simulink model "HarmonicDriveUr5_simulation"  (R2021a)
settings: Solver=ode15s  StartTime=0.0  StopTime=5  RelTol=1e-3
values from neighbouring files (symbols this model uses):
  K_lqr = lqr(A_c, B_c, Q, R)    [starterScript.m]
  Kd = 10    [starterScript.m]
  Ki = 2000    [starterScript.m]
  Kp = 40000    [starterScript.m]
  N = 100    [starterScript.m]
undefined symbols (not defined in the file or in its folder): X, Y, Z
libraries: fl_lib x60, sm_lib x57, nesl_utility x49, CustomComponents_lib x24, sdl_lib x6, roblocks x5
(part 1 of 3)
settings Model: Creator=agustin curri  LastModifiedBy=root
settings SolverCC: ZeroCrossAlgorithm=Adaptive  AlgebraicLoopSolver=TrustRegion
settings DebuggingCC: IgnoredZcDiagnostic=none  SFMachineParentedDataDiag=warning
settings ExplorerConfigSet: InternalSimMechanicsExplorerSettings="<ExplorerConfiguration><canonicalview>default</canonicalview><AnimationSetting><BasePlaybackSpeed>1.0</BasePlaybackSpeed><PlaybackSpeedFactor>1.0</PlaybackSpeedFactor></AnimationSetting><TilePanel><TileInfo><Tiles Columns=\"1\" Count=\"1\" Rows=\"1\"><Column Weight=\"1\"/><Row Weight=\"1\"/><Tile Height=\"1\" Width=\"1\" X=\"0\" Y=\"0\"/></Tiles></TileInfo><SceneInfo><SceneViewer><BGColor><R>1</R><G>1</G><B>1</B></BGColor><Camera><DoPerspective>off</DoPerspective><Position><X>0.024936801732020588</X><Y>-1.14355282845707174</Y><Z>0.464249949421630614</Z></Position><Center><X>0.024936801732020588</X><Y>-2.21862728744248727e-08</Y><Z>0.464249949421630614</Z></Center><Up><X>0</X><Y>-0</Y><Z>1</Z></Up><ViewLimDist>1</ViewLimDist><YLim>0.611217883330416378</YLim><XLim>1.22995074063620669</XLim></Camera></SceneViewer></SceneInfo></TilePanel><MechEditorPanel><Cameras/><GfxPanelCameraMap/><VideoCreator><PlaybackSpeedRatio>1.0</PlaybackSpeedRatio><FrameRate>30</FrameRate><VideoFormat>Motion JPEG AVI</VideoFormat><FrameSize>auto</FrameSize></VideoCreator></MechEditorPanel></ExplorerConfiguration>"

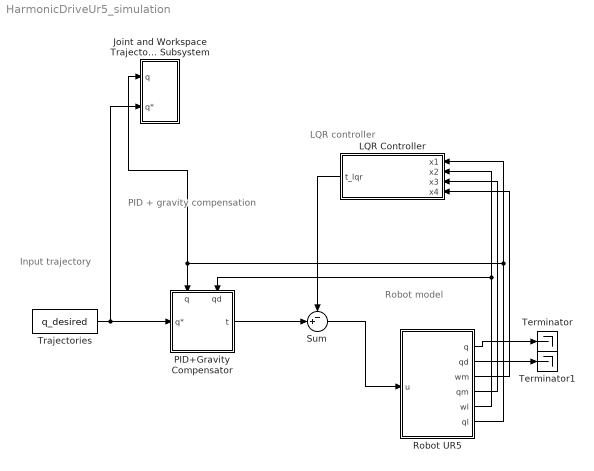
== system HarmonicDriveUr5_simulation ==
  note: Robot model
  note: LQR controller
  note: Input trajectory
  note: PID + gravity compensation
  Joint and Workspace Trajectory Subsystem : Subsystem
  LQR Controller : Subsystem
  PID+Gravity Compensator : Subsystem
      settings: PortSchema="{\"entries\":[{\"content\":{\"sides\":[{\"content\":{\"connectorIds\":[\"In1\"]},\"type\":\"ConnectorPlacement.EquallySpacedRectSide\",\"uuid\":\"10e36f8c-91af-4a0b-8edd-006e92f80377\"},{\"content\":{\"connectorIds\":[\"Out1\"],\"side\":\"RIGHT\"},\"type\":\"ConnectorPlacement.EquallySpacedRectSide\",\"uuid\":\"e975d4b2-2c07-4038-bb63-9e1fdc9bbfc2\"},{\"content\":{\"connectorIds\":[\"In2\",\"In3\"],\"side\":\"TOP\"},\"type\":\"ConnectorPlacement.EquallySpacedRectSide\",\"uuid\":\"401cadff-8190-4a51-9549-9161046c9efc\"}]},\"type\":\"ConnectorPlacement.EquallySpacedConnector\",\"uuid\":\"e3d6090e-dadc-41ed-ab00-96ae674af8f5\"}],\"packageUris\":[\"http://schema.mathworks.com/mf0/Connector/R2020b\"],\"version\":\"1.0\"}"
  Robot UR5 : Subsystem
  Sum : Sum  Inputs=-+|
  Terminator : Terminator
  Terminator1 : Terminator
  Trajectories : FromWorkspace  VariableName=q_desired
  wires:
  LQR Controller/1(t_lqr) -> Sum/1
  PID+Gravity Compensator/1(t) -> Sum/2
  Sum/1 -> Robot UR5/1(u)
  Trajectories/1 -> Joint and Workspace Trajectory Subsystem/2(q*), PID+Gravity Compensator/1(q*)
  Robot UR5/3(wm) -> LQR Controller/4(x4)
  Robot UR5/4(qm) -> LQR Controller/3(x3)
  Robot UR5/5(wl) -> PID+Gravity Compensator/3(qd), LQR Controller/2(x2)
  Robot UR5/6(ql) -> Joint and Workspace Trajectory Subsystem/1(q), PID+Gravity Compensator/2(q), LQR Controller/1(x1)
  Robot UR5/1(q) -> Terminator/1
  Robot UR5/2(qd) -> Terminator1/1

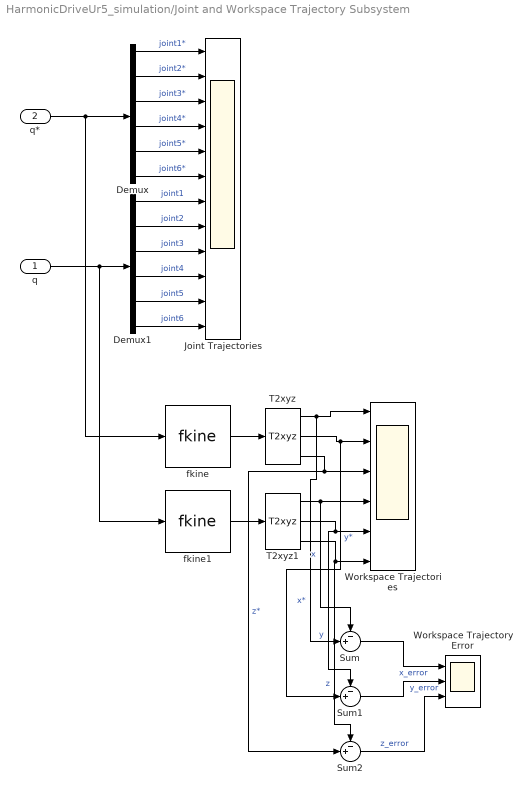
== system HarmonicDriveUr5_simulation/Joint and Workspace Trajectory Subsystem ==
  q : Inport
  q* : Inport  Port=2
  Demux : Demux  Outputs=6
  Demux1 : Demux  Outputs=6
  Joint Trajectories : Scope  NumInputPorts=12
  Sum : Sum  Inputs=-+|
  Sum1 : Sum  Inputs=-+|
  Sum2 : Sum  Inputs=-+|
  T2xyz : roblocks/Toolbox/T2xyz
  T2xyz1 : roblocks/Toolbox/T2xyz
  Workspace Trajectories : Scope  NumInputPorts=6
  Workspace Trajectory Error : Scope  NumInputPorts=3
  fkine : roblocks/Arm/fkine  robot=ur5
  fkine1 : roblocks/Arm/fkine  robot=ur5
  wires:
  Demux/4 -> Joint Trajectories/4  "joint4*"
  Demux1/2 -> Joint Trajectories/8  "joint2"
  Demux1/4 -> Joint Trajectories/10  "joint4"
  Demux1/6 -> Joint Trajectories/12  "joint6"
  Demux1/3 -> Joint Trajectories/9  "joint3"
  Demux/5 -> Joint Trajectories/5  "joint5*"
  Demux1/5 -> Joint Trajectories/11  "joint5"
  q*/1 -> fkine/1, Demux/1
  Demux/1 -> Joint Trajectories/1  "joint1*"
  q/1 -> fkine1/1, Demux1/1
  Demux1/1 -> Joint Trajectories/7  "joint1"
  Demux/6 -> Joint Trajectories/6  "joint6*"
  Demux/3 -> Joint Trajectories/3  "joint3*"
  Demux/2 -> Joint Trajectories/2  "joint2*"
  fkine/1 -> T2xyz/1
  T2xyz/1 -> Sum/2, Workspace Trajectories/1  "x*"
  T2xyz/2 -> Sum1/2, Workspace Trajectories/2  "y*"
  T2xyz/3 -> Workspace Trajectories/3, Sum2/2  "z*"
  fkine1/1 -> T2xyz1/1
  T2xyz1/1 -> Workspace Trajectories/4, Sum/1  "x"
  T2xyz1/2 -> Workspace Trajectories/5, Sum1/1  "y"
  T2xyz1/3 -> Workspace Trajectories/6, Sum2/1  "z"
  Sum/1 -> Workspace Trajectory Error/1  "x_error"
  Sum1/1 -> Workspace Trajectory Error/2  "y_error"
  Sum2/1 -> Workspace Trajectory Error/3  "z_error"

== system HarmonicDriveUr5_simulation/LQR Controller ==
  x1 : Inport
  x2 : Inport  Port=2
  x3 : Inport  Port=3
  x4 : Inport  Port=4
  MATLAB Function : MATLAB Function  TreatAsAtomicUnit=on  mask{K_lqr=K_lqr}
  Vector Concatenate : Concatenate  NumInputs=4
  t_lqr : Outport
  wires:
  x3/1 -> Vector Concatenate/3
  MATLAB Function/1(t) -> t_lqr/1
  Vector Concatenate/1 -> MATLAB Function/1(x)
  x1/1 -> Vector Concatenate/1
  x2/1 -> Vector Concatenate/2
  x4/1 -> Vector Concatenate/4

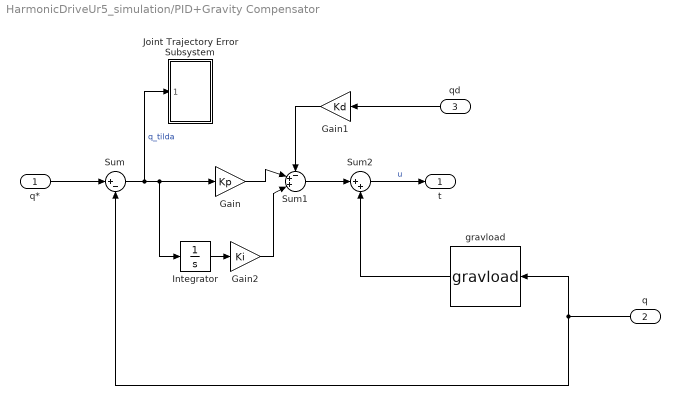
== system HarmonicDriveUr5_simulation/PID+Gravity Compensator ==
  q* : Inport
  q : Inport  Port=2
  qd : Inport  Port=3
  Gain : Gain  Gain=Kp
  Gain1 : Gain  Gain=Kd
  Gain2 : Gain  Gain=Ki
  Integrator : Integrator
  Joint Trajectory Error Subsystem : Subsystem
  Sum : Sum  Inputs=|+-
  Sum1 : Sum  Inputs=-++|
  Sum2 : Sum  Inputs=|++
  gravload : roblocks/Arm/gravload  robot=ur5
  t : Outport
  wires:
  Sum1/1 -> Sum2/1
  Sum/1 -> Joint Trajectory Error Subsystem/1(q_tilda), Gain/1, Integrator/1  "q_tilda"
  Gain2/1 -> Sum1/3
  qd/1 -> Gain1/1
  Integrator/1 -> Gain2/1
  q*/1 -> Sum/1
  q/1 -> gravload/1, Sum/2
  Gain1/1 -> Sum1/1
  Sum2/1 -> t/1  "u"
  Gain/1 -> Sum1/2
  gravload/1 -> Sum2/2

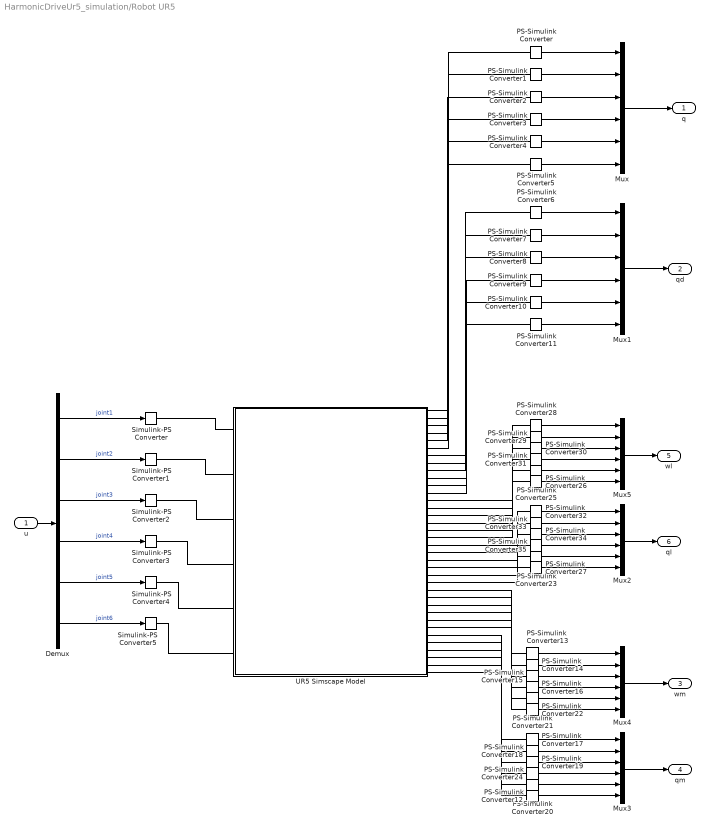
== system HarmonicDriveUr5_simulation/Robot UR5 ==
  u : Inport
  Demux : Demux  Outputs=6
  Mux{,1..5} (6 alike) : Mux  Inputs=6
  PS-Simulink Converter{,1..11} (12 alike) : nesl_utility/PS-Simulink Converter  PhysicalDomain=network_engine_domain  SubClassName=ps_output  LeftPortType=input  RightPortType=output  PseudoPeriodic=off  Frequencies=[]  Unit=inherit  AffineConversion=off
      settings: SourceProductBaseCode=PW,SS
  PS-Simulink Converter{12,17..20,23..24,27,32..35} (12 alike) : nesl_utility/PS-Simulink Converter  PhysicalDomain=network_engine_domain  SubClassName=ps_output  LeftPortType=input  RightPortType=output  PseudoPeriodic=off  Frequencies=[]  Unit=rad  AffineConversion=off
      settings: SourceProductBaseCode=PW,SS
  PS-Simulink Converter{13..16,21..22,25..26,28..31} (12 alike) : nesl_utility/PS-Simulink Converter  PhysicalDomain=network_engine_domain  SubClassName=ps_output  LeftPortType=input  RightPortType=output  PseudoPeriodic=off  Frequencies=[]  Unit=rad/s  AffineConversion=off
      settings: SourceProductBaseCode=PW,SS
  Simulink-PS Converter{,1..5} (6 alike) : nesl_utility/Simulink-PS Converter  PhysicalDomain=network_engine_domain  SubClassName=ps_input  LeftPortType=input  RightPortType=output  PseudoPeriodic=off  Frequencies=[]  NoiseDistribution=none  NoiseParameters=[]  Unit=1  AffineConversion=off  FilteringAndDerivatives=provide  SimscapeFilterOrder=2  InputFilterTimeConstant=0.001  UdotUserProvided=0
      settings: SourceProductBaseCode=PW,SS
  UR5 Simscape Model : Subsystem
  q : Outport
  qd : Outport  Port=2
  wm : Outport  Port=3
  qm : Outport  Port=4
  wl : Outport  Port=5
  ql : Outport  Port=6
  wires:
  Demux/6 -> Simulink-PS Converter5/1  "joint6"
  PS-Simulink Converter6/1 -> Mux1/1
  PS-Simulink Converter5/1 -> Mux/6
  PS-Simulink Converter7/1 -> Mux1/2
  PS-Simulink Converter8/1 -> Mux1/3
  u/1 -> Demux/1
  PS-Simulink Converter10/1 -> Mux1/5
  Demux/2 -> Simulink-PS Converter1/1  "joint2"
  PS-Simulink Converter4/1 -> Mux/5
  PS-Simulink Converter1/1 -> Mux/2
  PS-Simulink Converter/1 -> Mux/1
  Demux/1 -> Simulink-PS Converter/1  "joint1"
  Mux/1 -> q/1
  PS-Simulink Converter9/1 -> Mux1/4
  Mux1/1 -> qd/1
  Demux/5 -> Simulink-PS Converter4/1  "joint5"
  PS-Simulink Converter11/1 -> Mux1/6
  PS-Simulink Converter3/1 -> Mux/4
  Demux/4 -> Simulink-PS Converter3/1  "joint4"
  Demux/3 -> Simulink-PS Converter2/1  "joint3"
  PS-Simulink Converter2/1 -> Mux/3
  PS-Simulink Converter17/1 -> Mux3/1
  Mux3/1 -> qm/1
  PS-Simulink Converter18/1 -> Mux3/2
  PS-Simulink Converter14/1 -> Mux4/2
  PS-Simulink Converter15/1 -> Mux4/3
  PS-Simulink Converter13/1 -> Mux4/1
  PS-Simulink Converter21/1 -> Mux4/5
  PS-Simulink Converter24/1 -> Mux3/4
  PS-Simulink Converter20/1 -> Mux3/5
  PS-Simulink Converter12/1 -> Mux3/6
  PS-Simulink Converter19/1 -> Mux3/3
  PS-Simulink Converter22/1 -> Mux4/6
  PS-Simulink Converter16/1 -> Mux4/4
  Mux4/1 -> wm/1
  Mux5/1 -> wl/1
  PS-Simulink Converter26/1 -> Mux5/6
  PS-Simulink Converter29/1 -> Mux5/2
  PS-Simulink Converter31/1 -> Mux5/4
  PS-Simulink Converter25/1 -> Mux5/5
  Mux2/1 -> ql/1
  PS-Simulink Converter23/1 -> Mux2/5
  PS-Simulink Converter28/1 -> Mux5/1
  PS-Simulink Converter33/1 -> Mux2/2
  PS-Simulink Converter35/1 -> Mux2/4
  PS-Simulink Converter27/1 -> Mux2/6
  PS-Simulink Converter34/1 -> Mux2/3
  PS-Simulink Converter30/1 -> Mux5/3
  PS-Simulink Converter32/1 -> Mux2/1
  connections:
  UR5 Simscape Model/RConn1 -- PS-Simulink Converter/LConn1
  UR5 Simscape Model/RConn2 -- PS-Simulink Converter1/LConn1
  UR5 Simscape Model/RConn3 -- PS-Simulink Converter2/LConn1
  UR5 Simscape Model/RConn4 -- PS-Simulink Converter3/LConn1
  UR5 Simscape Model/RConn5 -- PS-Simulink Converter4/LConn1
  UR5 Simscape Model/RConn6 -- PS-Simulink Converter5/LConn1
  Simulink-PS Converter/RConn1 -- UR5 Simscape Model/LConn1
  UR5 Simscape Model/RConn7 -- PS-Simulink Converter6/LConn1
  Simulink-PS Converter1/RConn1 -- UR5 Simscape Model/LConn2
  UR5 Simscape Model/RConn8 -- PS-Simulink Converter7/LConn1
  Simulink-PS Converter2/RConn1 -- UR5 Simscape Model/LConn3
  UR5 Simscape Model/RConn9 -- PS-Simulink Converter8/LConn1
  Simulink-PS Converter3/RConn1 -- UR5 Simscape Model/LConn4
  UR5 Simscape Model/RConn10 -- PS-Simulink Converter9/LConn1
  Simulink-PS Converter4/RConn1 -- UR5 Simscape Model/LConn5
  UR5 Simscape Model/RConn11 -- PS-Simulink Converter10/LConn1
  Simulink-PS Converter5/RConn1 -- UR5 Simscape Model/LConn6
  UR5 Simscape Model/RConn12 -- PS-Simulink Converter11/LConn1
  UR5 Simscape Model/RConn25 -- PS-Simulink Converter13/LConn1
  UR5 Simscape Model/RConn26 -- PS-Simulink Converter14/LConn1
  UR5 Simscape Model/RConn27 -- PS-Simulink Converter15/LConn1
  UR5 Simscape Model/RConn28 -- PS-Simulink Converter16/LConn1
  UR5 Simscape Model/RConn29 -- PS-Simulink Converter21/LConn1
  UR5 Simscape Model/RConn30 -- PS-Simulink Converter22/LConn1
  UR5 Simscape Model/RConn31 -- PS-Simulink Converter17/LConn1
  UR5 Simscape Model/RConn32 -- PS-Simulink Converter18/LConn1
  UR5 Simscape Model/RConn33 -- PS-Simulink Converter19/LConn1
  UR5 Simscape Model/RConn34 -- PS-Simulink Converter24/LConn1
  UR5 Simscape Model/RConn35 -- PS-Simulink Converter20/LConn1
  UR5 Simscape Model/RConn36 -- PS-Simulink Converter12/LConn1
  UR5 Simscape Model/RConn13 -- PS-Simulink Converter28/LConn1
  UR5 Simscape Model/RConn14 -- PS-Simulink Converter29/LConn1
  UR5 Simscape Model/RConn15 -- PS-Simulink Converter30/LConn1
  UR5 Simscape Model/RConn16 -- PS-Simulink Converter31/LConn1
  UR5 Simscape Model/RConn17 -- PS-Simulink Converter25/LConn1
  UR5 Simscape Model/RConn18 -- PS-Simulink Converter26/LConn1
  UR5 Simscape Model/RConn19 -- PS-Simulink Converter32/LConn1
  UR5 Simscape Model/RConn20 -- PS-Simulink Converter33/LConn1
  UR5 Simscape Model/RConn21 -- PS-Simulink Converter34/LConn1
  UR5 Simscape Model/RConn22 -- PS-Simulink Converter35/LConn1
  UR5 Simscape Model/RConn23 -- PS-Simulink Converter23/LConn1
  UR5 Simscape Model/RConn24 -- PS-Simulink Converter27/LConn1

== system HarmonicDriveUr5_simulation/PID+Gravity Compensator/Joint Trajectory Error Subsystem ==
  q_tilda : Inport
  Demux : Demux  Outputs=6
  Joint Trajectory Error : Scope  NumInputPorts=6
  wires:
  Demux/5 -> Joint Trajectory Error/5  "joint5"
  q_tilda/1 -> Demux/1
  Demux/2 -> Joint Trajectory Error/2  "joint2"
  Demux/3 -> Joint Trajectory Error/3  "joint3"
  Demux/4 -> Joint Trajectory Error/4  "joint4"
  Demux/6 -> Joint Trajectory Error/6  "joint6"
  Demux/1 -> Joint Trajectory Error/1  "joint1"

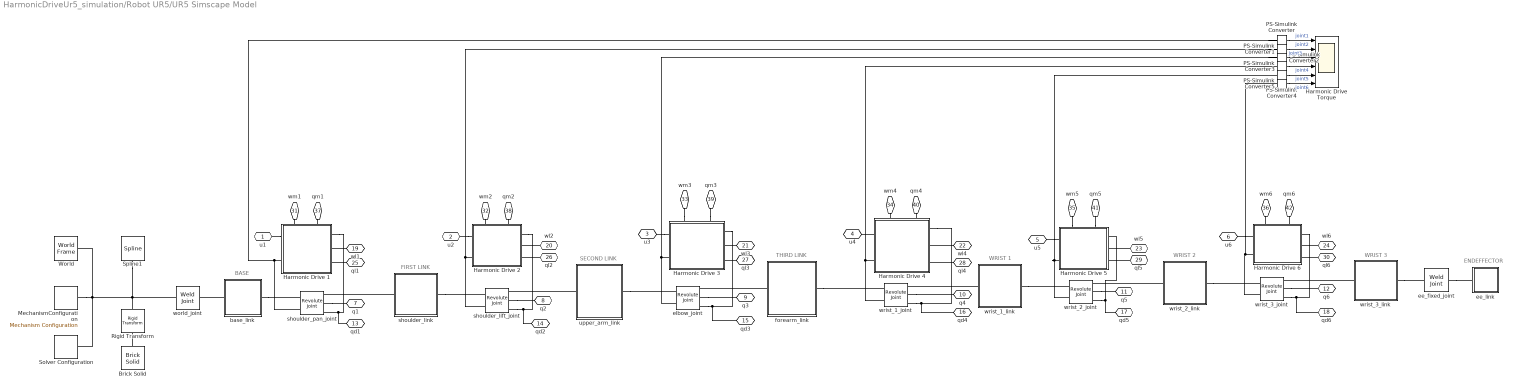
== system HarmonicDriveUr5_simulation/Robot UR5/UR5 Simscape Model ==
  note: BASE
  note: FIRST LINK
  note: SECOND LINK
  note: THIRD LINK
  note: WRIST 1
  note: WRIST 2
  note: WRIST 3
  note: ENDEFFECTOR
  Brick Solid : sm_lib/Body Elements/Brick Solid  GraphicAmbientColor=[0.15 0.15 0.15 1.0]  BasedOnType=Density  BrickDimensions=[.5 .5 0.2]  BrickDimensionUnits=m  CenterOfMass=[0 0 0]  CenterOfMassUnits=m  GraphicDiffuseColor=[0.8 1.0 0.6]  Density=1000  DensityUnits=kg/m^3  DoExposeReferenceFrame=on  GraphicEmissiveColor=[0.0 0.0 0.0 1.0]  ExportEntireGeometry=off  SerializedFrames=<Frames/>  MarkerShape=Sphere  MarkerSize=10  GraphicType=FromGeometry  InertiaType=CalculateFromGeometry  Mass=1  MassUnits=kg  MomentsOfInertia=[1 1 1]  MomentsOfInertiaUnits=kg*m^2  GraphicOpacity=1.0  ProductsOfInertia=[0 0 0]  ProductsOfInertiaUnits=kg*m^2  GraphicShininess=75  GraphicSpecularColor=[0.5 0.5 0.5 1.0]  GraphicVisPropType=SimpleVisualProperties
  Harmonic Drive 1 : Subsystem
      settings: PortSchema="{\"entries\":[{\"content\":{\"sides\":[{\"content\":{\"connectorIds\":[\"LConn1\",\"LConn2\"]},\"type\":\"ConnectorPlacement.EquallySpacedRectSide\",\"uuid\":\"507705ac-a0fa-4fe7-8f73-31050ecbd987\"},{\"content\":{\"connectorIds\":[\"RConn1\",\"RConn2\",\"RConn3\"],\"side\":\"RIGHT\"},\"type\":\"ConnectorPlacement.EquallySpacedRectSide\",\"uuid\":\"f13bfcdd-63e8-47b4-aefd-dba91edbc643\"},{\"content\":{\"connectorIds\":[\"LConn3\",\"LConn4\"],\"side\":\"TOP\"},\"type\":\"ConnectorPlacement.EquallySpacedRectSide\",\"uuid\":\"144ffa6a-f599-4bcb-ae05-6789f1cae58f\"}]},\"type\":\"ConnectorPlacement.EquallySpacedConnector\",\"uuid\":\"4d436d19-1cb5-4db6-9907-e987ea85be45\"}],\"packageUris\":[\"http://schema.mathworks.com/mf0/Connector/R2020b\"],\"version\":\"1.0\"}"
      mask Display: image('$imagefile'); % Use "Edit Image" on toolstrip to change.
  Harmonic Drive 2 : Subsystem
      settings: PortSchema="{\"entries\":[{\"content\":{\"sides\":[{\"content\":{\"connectorIds\":[\"LConn1\",\"LConn2\"]},\"type\":\"ConnectorPlacement.EquallySpacedRectSide\",\"uuid\":\"507705ac-a0fa-4fe7-8f73-31050ecbd987\"},{\"content\":{\"connectorIds\":[\"RConn1\",\"RConn2\",\"RConn3\"],\"side\":\"RIGHT\"},\"type\":\"ConnectorPlacement.EquallySpacedRectSide\",\"uuid\":\"f13bfcdd-63e8-47b4-aefd-dba91edbc643\"},{\"content\":{\"connectorIds\":[\"LConn3\",\"LConn4\"],\"side\":\"TOP\"},\"type\":\"ConnectorPlacement.EquallySpacedRectSide\",\"uuid\":\"144ffa6a-f599-4bcb-ae05-6789f1cae58f\"}]},\"type\":\"ConnectorPlacement.EquallySpacedConnector\",\"uuid\":\"4d436d19-1cb5-4db6-9907-e987ea85be45\"}],\"packageUris\":[\"http://schema.mathworks.com/mf0/Connector/R2020b\"],\"version\":\"1.0\"}"
      mask Display: image('$imagefile'); % Use "Edit Image" on toolstrip to change.
  Harmonic Drive 3 : Subsystem
      settings: PortSchema="{\"entries\":[{\"content\":{\"sides\":[{\"content\":{\"connectorIds\":[\"LConn1\",\"LConn2\"]},\"type\":\"ConnectorPlacement.EquallySpacedRectSide\",\"uuid\":\"507705ac-a0fa-4fe7-8f73-31050ecbd987\"},{\"content\":{\"connectorIds\":[\"RConn1\",\"RConn2\",\"RConn3\"],\"side\":\"RIGHT\"},\"type\":\"ConnectorPlacement.EquallySpacedRectSide\",\"uuid\":\"f13bfcdd-63e8-47b4-aefd-dba91edbc643\"},{\"content\":{\"connectorIds\":[\"LConn3\",\"LConn4\"],\"side\":\"TOP\"},\"type\":\"ConnectorPlacement.EquallySpacedRectSide\",\"uuid\":\"144ffa6a-f599-4bcb-ae05-6789f1cae58f\"}]},\"type\":\"ConnectorPlacement.EquallySpacedConnector\",\"uuid\":\"4d436d19-1cb5-4db6-9907-e987ea85be45\"}],\"packageUris\":[\"http://schema.mathworks.com/mf0/Connector/R2020b\"],\"version\":\"1.0\"}"
      mask Display: image('$imagefile'); % Use "Edit Image" on toolstrip to change.
  Harmonic Drive 4 : Subsystem
      settings: PortSchema="{\"entries\":[{\"content\":{\"sides\":[{\"content\":{\"connectorIds\":[\"LConn1\",\"LConn2\"]},\"type\":\"ConnectorPlacement.EquallySpacedRectSide\",\"uuid\":\"507705ac-a0fa-4fe7-8f73-31050ecbd987\"},{\"content\":{\"connectorIds\":[\"RConn1\",\"RConn2\",\"RConn3\"],\"side\":\"RIGHT\"},\"type\":\"ConnectorPlacement.EquallySpacedRectSide\",\"uuid\":\"f13bfcdd-63e8-47b4-aefd-dba91edbc643\"},{\"content\":{\"connectorIds\":[\"LConn3\",\"LConn4\"],\"side\":\"TOP\"},\"type\":\"ConnectorPlacement.EquallySpacedRectSide\",\"uuid\":\"144ffa6a-f599-4bcb-ae05-6789f1cae58f\"}]},\"type\":\"ConnectorPlacement.EquallySpacedConnector\",\"uuid\":\"4d436d19-1cb5-4db6-9907-e987ea85be45\"}],\"packageUris\":[\"http://schema.mathworks.com/mf0/Connector/R2020b\"],\"version\":\"1.0\"}"
      mask Display: image('$imagefile'); % Use "Edit Image" on toolstrip to change.
  Harmonic Drive 5 : Subsystem
      settings: PortSchema="{\"entries\":[{\"content\":{\"sides\":[{\"content\":{\"connectorIds\":[\"LConn1\",\"LConn2\"]},\"type\":\"ConnectorPlacement.EquallySpacedRectSide\",\"uuid\":\"507705ac-a0fa-4fe7-8f73-31050ecbd987\"},{\"content\":{\"connectorIds\":[\"RConn1\",\"RConn2\",\"RConn3\"],\"side\":\"RIGHT\"},\"type\":\"ConnectorPlacement.EquallySpacedRectSide\",\"uuid\":\"f13bfcdd-63e8-47b4-aefd-dba91edbc643\"},{\"content\":{\"connectorIds\":[\"LConn3\",\"LConn4\"],\"side\":\"TOP\"},\"type\":\"ConnectorPlacement.EquallySpacedRectSide\",\"uuid\":\"144ffa6a-f599-4bcb-ae05-6789f1cae58f\"}]},\"type\":\"ConnectorPlacement.EquallySpacedConnector\",\"uuid\":\"4d436d19-1cb5-4db6-9907-e987ea85be45\"}],\"packageUris\":[\"http://schema.mathworks.com/mf0/Connector/R2020b\"],\"version\":\"1.0\"}"
      mask Display: image('$imagefile'); % Use "Edit Image" on toolstrip to change.
  Harmonic Drive 6 : Subsystem
      settings: PortSchema="{\"entries\":[{\"content\":{\"sides\":[{\"content\":{\"connectorIds\":[\"LConn1\",\"LConn2\"]},\"type\":\"ConnectorPlacement.EquallySpacedRectSide\",\"uuid\":\"507705ac-a0fa-4fe7-8f73-31050ecbd987\"},{\"content\":{\"connectorIds\":[\"RConn1\",\"RConn2\",\"RConn3\"],\"side\":\"RIGHT\"},\"type\":\"ConnectorPlacement.EquallySpacedRectSide\",\"uuid\":\"f13bfcdd-63e8-47b4-aefd-dba91edbc643\"},{\"content\":{\"connectorIds\":[\"LConn3\",\"LConn4\"],\"side\":\"TOP\"},\"type\":\"ConnectorPlacement.EquallySpacedRectSide\",\"uuid\":\"144ffa6a-f599-4bcb-ae05-6789f1cae58f\"}]},\"type\":\"ConnectorPlacement.EquallySpacedConnector\",\"uuid\":\"4d436d19-1cb5-4db6-9907-e987ea85be45\"}],\"packageUris\":[\"http://schema.mathworks.com/mf0/Connector/R2020b\"],\"version\":\"1.0\"}"
      mask Display: image('$imagefile'); % Use "Edit Image" on toolstrip to change.
  Harmonic Drive Torque : Scope  NumInputPorts=6
  MechanismConfiguration : sm_lib/Utilities/Mechanism Configuration  UniformGravity=Constant  GravityVector=[0 0 -9.80665]  GravityVectorUnits=m/s^2  GravityUnits=m/s^2  LinearizationDelta=0.001  JointModeTransitionNonlinearIterations=2
  PS-Simulink Converter{,1..5} (6 alike) : nesl_utility/PS-Simulink Converter  PhysicalDomain=network_engine_domain  SubClassName=ps_output  LeftPortType=input  RightPortType=output  PseudoPeriodic=off  Frequencies=[]  Unit=inherit  AffineConversion=off
      settings: SourceProductBaseCode=PW,SS
  Rigid Transform : sm_lib/Frames and Transforms/Rigid Transform  TranslationMethod=Cartesian  TranslationStandardOffset=0  TranslationLengthUnit=m  TranslationStandardAxis=+Z  TranslationCartesianOffset=[0 0 0.1]  TranslationROffset=0  TranslationROffsetUnits=m  TranslationZOffset=0  TranslationZOffsetUnits=m  TranslationThetaOffset=0  TranslationThetaOffsetUnits=deg  RotationMethod=None  RotationAngleUnits=deg  RotationStandardAxis=+Z  RotationAngle=0.0  RotationArbitraryAxis=[0 0 1]  FollAlignAxisA=+X  BaseAlignAxisA=+Y  FollAlignAxisB=+Y  BaseAlignAxisB=+Z  RotationSequenceAxes=FollowerAxes  RotationSequence=XYX  RotationSequenceAngles=[0 0 0]  RotationSequenceAnglesUnits=deg  RotationMatrix=[1 0 0; 0 1 0; 0 0 1]
  Solver Configuration : nesl_utility/Solver Configuration  PhysicalDomain=network_engine_domain  SubClassName=solver  LeftPortType=input  RightPortType=generic  Tones=[]  Harmonics=[]  SimulateNoise=off  Profile=off  UseLocalSampling=off  EnableSwitchedLinearOptims=on  FrequencyDomain=off  UseCCode=off  RelTol=0.001  AbsTol=1e-06  MinStep=1e-09  ToWorkspace=off  RevertToSquareIcSolve=off  NumHomotopyIterations=100  PhasorMode=off  PhasorModeNumHarmonics=1  DoDC=off  ResidualTolerance=1e-09  UseLocalSolver=off  LocalSolverChoice=NE_BACKWARD_EULER_ADVANCER  LocalSolverSampleTime=0.001  DoFixedCost=off  MaxNonlinIter=3  MaxModeIter=2  ComputeImpulses=off  ImpulseIterations=2  LinearAlgebra=auto  EquationFormulation=NE_TIME_EF  DelaysMemoryBudget=1024  AutomaticFiltering=on  FilteringTimeConstant=0.001  PartitionStorageMethod=AS_NEEDED  PartitionMemoryBudget=1024  PartitionMethod=ROBUST
      settings: SourceProductBaseCode=PW,SS
  Spline1 : sm_lib/Curves and Surfaces/Spline  GraphicAmbientColor=[0.15 0.15 0.15 1.0]  GraphicDiffuseColor=[0.0 0.0 0.8]  DataPoints=traj_visual  DataPointsUnits=m  GraphicEmissiveColor=[0.0 0.0 0.0 1.0]  EndConditionType=Natural  MarkerShape=Sphere  MarkerSize=10  GraphicType=FromGeometry  GraphicOpacity=1.0  GraphicShininess=75  GraphicSpecularColor=[0.5 0.5 0.5 1.0]  GraphicVisPropType=SimpleVisualProperties
  World : sm_lib/Frames and Transforms/World Frame
  base_link : Subsystem
  ee_fixed_joint : sm_lib/Joints/Weld Joint  JointMode=Normal  SenseConstraintForce=off  SenseConstraintForceX=off  SenseConstraintForceY=off  SenseConstraintForceZ=off  SenseConstraintTorque=off  SenseConstraintTorqueX=off  SenseConstraintTorqueY=off  SenseConstraintTorqueZ=off  SenseTotalForce=off  SenseTotalForceX=off  SenseTotalForceY=off  SenseTotalForceZ=off  SenseTotalTorque=off  SenseTotalTorqueX=off  SenseTotalTorqueY=off  SenseTotalTorqueZ=off  CompositeWrenchDir=FollowerOnBase  CompositeWrenchFrame=BaseFrame
  ee_link : Subsystem
  elbow_joint : sm_lib/Joints/Revolute Joint  JointMode=Normal  SenseConstraintForce=off  SenseConstraintForceX=off  SenseConstraintForceY=off  SenseConstraintForceZ=off  SenseConstraintTorque=off  SenseConstraintTorqueX=off  SenseConstraintTorqueY=off  SenseConstraintTorqueZ=off  SenseTotalForce=off  SenseTotalForceX=off  SenseTotalForceY=off  SenseTotalForceZ=off  SenseTotalTorque=off  SenseTotalTorqueX=off  SenseTotalTorqueY=off  SenseTotalTorqueZ=off  CompositeWrenchDir=FollowerOnBase  CompositeWrenchFrame=BaseFrame  EquilibriumPosition=0  EquilibriumPositionUnits=deg  SpringStiffness=0  SpringStiffnessUnits=N*m/deg  DampingCoefficient=0  DampingCoefficientUnits=m^2*kg/s/rad  TorqueActuationMode=InputTorque  MotionActuationMode=ComputedMotion  SensePosition=on  SenseVelocity=on  SenseAcceleration=off  SenseTorqueForce=off  SenseLowerLimitTorqueForce=off  SenseUpperLimitTorqueForce=off  LowerLimitSpecify=on  LowerLimitBound=-6.2831853  LowerLimitBoundUnits=rad  LowerLimitStiffness=1e4  LowerLimitStiffnessUnits=N*m/deg  LowerLimitDamping=10  LowerLimitDampingUnits=N*m/(deg/s)  LowerLimitTransitionRegionWidth=0.1  LowerLimitTransitionRegionWidthUnits=deg  UpperLimitSpecify=on  UpperLimitBound=6.2831853  UpperLimitBoundUnits=rad  UpperLimitStiffness=1e4  UpperLimitStiffnessUnits=N*m/deg  UpperLimitDamping=10  UpperLimitDampingUnits=N*m/(deg/s)  UpperLimitTransitionRegionWidth=0.1  UpperLimitTransitionRegionWidthUnits=deg  PositionTargetSpecify=off  PositionTargetPriority=High  PositionTargetValue=0.998709954143429  PositionTargetValueUnits=rad  VelocityTargetSpecify=off  VelocityTargetPriority=High  VelocityTargetValue=0  VelocityTargetValueUnits=deg/s
  forearm_link : Subsystem
  shoulder_lift_joint : sm_lib/Joints/Revolute Joint  JointMode=Normal  SenseConstraintForce=off  SenseConstraintForceX=off  SenseConstraintForceY=off  SenseConstraintForceZ=off  SenseConstraintTorque=off  SenseConstraintTorqueX=off  SenseConstraintTorqueY=off  SenseConstraintTorqueZ=off  SenseTotalForce=off  SenseTotalForceX=off  SenseTotalForceY=off  SenseTotalForceZ=off  SenseTotalTorque=off  SenseTotalTorqueX=off  SenseTotalTorqueY=off  SenseTotalTorqueZ=off  CompositeWrenchDir=FollowerOnBase  CompositeWrenchFrame=BaseFrame  EquilibriumPosition=0  EquilibriumPositionUnits=deg  SpringStiffness=0  SpringStiffnessUnits=N*m/deg  DampingCoefficient=0  DampingCoefficientUnits=m^2*kg/s/rad  TorqueActuationMode=InputTorque  MotionActuationMode=ComputedMotion  SensePosition=on  SenseVelocity=on  SenseAcceleration=off  SenseTorqueForce=off  SenseLowerLimitTorqueForce=off  SenseUpperLimitTorqueForce=off  LowerLimitSpecify=on  LowerLimitBound=-6.2831853  LowerLimitBoundUnits=rad  LowerLimitStiffness=1e4  LowerLimitStiffnessUnits=N*m/deg  LowerLimitDamping=10  LowerLimitDampingUnits=N*m/(deg/s)  LowerLimitTransitionRegionWidth=0.1  LowerLimitTransitionRegionWidthUnits=deg  UpperLimitSpecify=on  UpperLimitBound=6.2831853  UpperLimitBoundUnits=rad  UpperLimitStiffness=1e4  UpperLimitStiffnessUnits=N*m/deg  UpperLimitDamping=10  UpperLimitDampingUnits=N*m/(deg/s)  UpperLimitTransitionRegionWidth=0.1  UpperLimitTransitionRegionWidthUnits=deg  PositionTargetSpecify=off  PositionTargetPriority=High  PositionTargetValue=-1.58863637968653  PositionTargetValueUnits=rad  VelocityTargetSpecify=off  VelocityTargetPriority=High  VelocityTargetValue=0  VelocityTargetValueUnits=deg/s
  shoulder_link : Subsystem
  shoulder_pan_joint : sm_lib/Joints/Revolute Joint  JointMode=Normal  SenseConstraintForce=off  SenseConstraintForceX=off  SenseConstraintForceY=off  SenseConstraintForceZ=off  SenseConstraintTorque=off  SenseConstraintTorqueX=off  SenseConstraintTorqueY=off  SenseConstraintTorqueZ=off  SenseTotalForce=off  SenseTotalForceX=off  SenseTotalForceY=off  SenseTotalForceZ=off  SenseTotalTorque=off  SenseTotalTorqueX=off  SenseTotalTorqueY=off  SenseTotalTorqueZ=off  CompositeWrenchDir=FollowerOnBase  CompositeWrenchFrame=BaseFrame  EquilibriumPosition=0  EquilibriumPositionUnits=deg  SpringStiffness=0  SpringStiffnessUnits=N*m/deg  DampingCoefficient=0  DampingCoefficientUnits=m^2*kg/s/rad  TorqueActuationMode=InputTorque  MotionActuationMode=ComputedMotion  SensePosition=on  SenseVelocity=on  SenseAcceleration=off  SenseTorqueForce=off  SenseLowerLimitTorqueForce=off  SenseUpperLimitTorqueForce=off  LowerLimitSpecify=on  LowerLimitBound=-6.2831853  LowerLimitBoundUnits=rad  LowerLimitStiffness=1e4  LowerLimitStiffnessUnits=N*m/deg  LowerLimitDamping=10  LowerLimitDampingUnits=N*m/(deg/s)  LowerLimitTransitionRegionWidth=0.1  LowerLimitTransitionRegionWidthUnits=deg  UpperLimitSpecify=on  UpperLimitBound=6.2831853  UpperLimitBoundUnits=rad  UpperLimitStiffness=1e4  UpperLimitStiffnessUnits=N*m/deg  UpperLimitDamping=10  UpperLimitDampingUnits=N*m/(deg/s)  UpperLimitTransitionRegionWidth=0.1  UpperLimitTransitionRegionWidthUnits=deg  PositionTargetSpecify=off  PositionTargetPriority=High  PositionTargetValue=2.52445629759502+pi  PositionTargetValueUnits=rad  VelocityTargetSpecify=off  VelocityTargetPriority=High  VelocityTargetValue=0  VelocityTargetValueUnits=deg/s
  upper_arm_link : Subsystem
  world_joint : sm_lib/Joints/Weld Joint  JointMode=Normal  SenseConstraintForce=off  SenseConstraintForceX=off  SenseConstraintForceY=off  SenseConstraintForceZ=off  SenseConstraintTorque=off  SenseConstraintTorqueX=off  SenseConstraintTorqueY=off  SenseConstraintTorqueZ=off  SenseTotalForce=off  SenseTotalForceX=off  SenseTotalForceY=off  SenseTotalForceZ=off  SenseTotalTorque=off  SenseTotalTorqueX=off  SenseTotalTorqueY=off  SenseTotalTorqueZ=off  CompositeWrenchDir=FollowerOnBase  CompositeWrenchFrame=BaseFrame
  wrist_1_joint : sm_lib/Joints/Revolute Joint  JointMode=Normal  SenseConstraintForce=off  SenseConstraintForceX=off  SenseConstraintForceY=off  SenseConstraintForceZ=off  SenseConstraintTorque=off  SenseConstraintTorqueX=off  SenseConstraintTorqueY=off  SenseConstraintTorqueZ=off  SenseTotalForce=off  SenseTotalForceX=off  SenseTotalForceY=off  SenseTotalForceZ=off  SenseTotalTorque=off  SenseTotalTorqueX=off  SenseTotalTorqueY=off  SenseTotalTorqueZ=off  CompositeWrenchDir=FollowerOnBase  CompositeWrenchFrame=BaseFrame  EquilibriumPosition=0  EquilibriumPositionUnits=deg  SpringStiffness=0  SpringStiffnessUnits=N*m/deg  DampingCoefficient=0  DampingCoefficientUnits=m^2*kg/s/rad  TorqueActuationMode=InputTorque  MotionActuationMode=ComputedMotion  SensePosition=on  SenseVelocity=on  SenseAcceleration=off  SenseTorqueForce=off  SenseLowerLimitTorqueForce=off  SenseUpperLimitTorqueForce=off  LowerLimitSpecify=on  LowerLimitBound=-6.2831853  LowerLimitBoundUnits=rad  LowerLimitStiffness=1e4  LowerLimitStiffnessUnits=N*m/deg  LowerLimitDamping=10  LowerLimitDampingUnits=N*m/(deg/s)  LowerLimitTransitionRegionWidth=0.1  LowerLimitTransitionRegionWidthUnits=deg  UpperLimitSpecify=on  UpperLimitBound=6.2831853  UpperLimitBoundUnits=rad  UpperLimitStiffness=1e4  UpperLimitStiffnessUnits=N*m/deg  UpperLimitDamping=10  UpperLimitDampingUnits=N*m/(deg/s)  UpperLimitTransitionRegionWidth=0.1  UpperLimitTransitionRegionWidthUnits=deg  PositionTargetSpecify=off  PositionTargetPriority=High  PositionTargetValue=-0.980869901251790  PositionTargetValueUnits=rad  VelocityTargetSpecify=off  VelocityTargetPriority=High  VelocityTargetValue=0  VelocityTargetValueUnits=deg/s
  wrist_1_link : Subsystem
  wrist_2_joint : sm_lib/Joints/Revolute Joint  JointMode=Normal  SenseConstraintForce=off  SenseConstraintForceX=off  SenseConstraintForceY=off  SenseConstraintForceZ=off  SenseConstraintTorque=off  SenseConstraintTorqueX=off  SenseConstraintTorqueY=off  SenseConstraintTorqueZ=off  SenseTotalForce=off  SenseTotalForceX=off  SenseTotalForceY=off  SenseTotalForceZ=off  SenseTotalTorque=off  SenseTotalTorqueX=off  SenseTotalTorqueY=off  SenseTotalTorqueZ=off  CompositeWrenchDir=FollowerOnBase  CompositeWrenchFrame=BaseFrame  EquilibriumPosition=0  EquilibriumPositionUnits=deg  SpringStiffness=0  SpringStiffnessUnits=N*m/deg  DampingCoefficient=0  DampingCoefficientUnits=m^2*kg/s/rad  TorqueActuationMode=InputTorque  MotionActuationMode=ComputedMotion  SensePosition=on  SenseVelocity=on  SenseAcceleration=off  SenseTorqueForce=off  SenseLowerLimitTorqueForce=off  SenseUpperLimitTorqueForce=off  LowerLimitSpecify=on  LowerLimitBound=-6.2831853  LowerLimitBoundUnits=rad  LowerLimitStiffness=1e4  LowerLimitStiffnessUnits=N*m/deg  LowerLimitDamping=10  LowerLimitDampingUnits=N*m/(deg/s)  LowerLimitTransitionRegionWidth=0.1  LowerLimitTransitionRegionWidthUnits=deg  UpperLimitSpecify=on  UpperLimitBound=6.2831853  UpperLimitBoundUnits=rad  UpperLimitStiffness=1e4  UpperLimitStiffnessUnits=N*m/deg  UpperLimitDamping=10  UpperLimitDampingUnits=N*m/(deg/s)  UpperLimitTransitionRegionWidth=0.1  UpperLimitTransitionRegionWidthUnits=deg  PositionTargetSpecify=off  PositionTargetPriority=High  PositionTargetValue=-1.57079632679490  PositionTargetValueUnits=rad  VelocityTargetSpecify=off  VelocityTargetPriority=High  VelocityTargetValue=0  VelocityTargetValueUnits=deg/s
  wrist_2_link : Subsystem
  wrist_3_joint : sm_lib/Joints/Revolute Joint  JointMode=Normal  SenseConstraintForce=off  SenseConstraintForceX=off  SenseConstraintForceY=off  SenseConstraintForceZ=off  SenseConstraintTorque=off  SenseConstraintTorqueX=off  SenseConstraintTorqueY=off  SenseConstraintTorqueZ=off  SenseTotalForce=off  SenseTotalForceX=off  SenseTotalForceY=off  SenseTotalForceZ=off  SenseTotalTorque=off  SenseTotalTorqueX=off  SenseTotalTorqueY=off  SenseTotalTorqueZ=off  CompositeWrenchDir=FollowerOnBase  CompositeWrenchFrame=BaseFrame  EquilibriumPosition=0  EquilibriumPositionUnits=deg  SpringStiffness=0  SpringStiffnessUnits=N*m/deg  DampingCoefficient=0  DampingCoefficientUnits=m^2*kg/s/rad  TorqueActuationMode=InputTorque  MotionActuationMode=ComputedMotion  SensePosition=on  SenseVelocity=on  SenseAcceleration=off  SenseTorqueForce=off  SenseLowerLimitTorqueForce=off  SenseUpperLimitTorqueForce=off  LowerLimitSpecify=on  LowerLimitBound=-6.2831853  LowerLimitBoundUnits=rad  LowerLimitStiffness=1e4  LowerLimitStiffnessUnits=N*m/deg  LowerLimitDamping=10  LowerLimitDampingUnits=N*m/(deg/s)  LowerLimitTransitionRegionWidth=0.1  LowerLimitTransitionRegionWidthUnits=deg  UpperLimitSpecify=on  UpperLimitBound=6.2831853  UpperLimitBoundUnits=rad  UpperLimitStiffness=1e4  UpperLimitStiffnessUnits=N*m/deg  UpperLimitDamping=10  UpperLimitDampingUnits=N*m/(deg/s)  UpperLimitTransitionRegionWidth=0.1  UpperLimitTransitionRegionWidthUnits=deg  PositionTargetSpecify=off  PositionTargetPriority=High  PositionTargetValue=2.52445629759502  PositionTargetValueUnits=rad  VelocityTargetSpecify=off  VelocityTargetPriority=High  VelocityTargetValue=0  VelocityTargetValueUnits=deg/s
  wrist_3_link : Subsystem
  u1 : PMIOPort  Side=Left
  u2 : PMIOPort  Port=2  Side=Left
  u3 : PMIOPort  Port=3  Side=Left
  u4 : PMIOPort  Port=4  Side=Left
  u5 : PMIOPort  Port=5  Side=Left
  u6 : PMIOPort  Port=6  Side=Left
  q1 : PMIOPort  Port=7  Side=Right
  q2 : PMIOPort  Port=8  Side=Right
  q3 : PMIOPort  Port=9  Side=Right
  q4 : PMIOPort  Port=10  Side=Right
  q5 : PMIOPort  Port=11  Side=Right
  q6 : PMIOPort  Port=12  Side=Right
  qd1 : PMIOPort  Port=13  Side=Right
  qd2 : PMIOPort  Port=14  Side=Right
  qd3 : PMIOPort  Port=15  Side=Right
  qd4 : PMIOPort  Port=16  Side=Right
  qd5 : PMIOPort  Port=17  Side=Right
  qd6 : PMIOPort  Port=18  Side=Right
  wl1 : PMIOPort  Port=19  Side=Right
  wl2 : PMIOPort  Port=20  Side=Right
  wl3 : PMIOPort  Port=21  Side=Right
  wl4 : PMIOPort  Port=22  Side=Right
  wl5 : PMIOPort  Port=23  Side=Right
  wl6 : PMIOPort  Port=24  Side=Right
  ql1 : PMIOPort  Port=25  Side=Right
  ql2 : PMIOPort  Port=26  Side=Right
  ql3 : PMIOPort  Port=27  Side=Right
  ql4 : PMIOPort  Port=28  Side=Right
  ql5 : PMIOPort  Port=29  Side=Right
  ql6 : PMIOPort  Port=30  Side=Right
  wm1 : PMIOPort  Port=31  Side=Right
  wm2 : PMIOPort  Port=32  Side=Right
  wm3 : PMIOPort  Port=33  Side=Right
  wm4 : PMIOPort  Port=34  Side=Right
  wm5 : PMIOPort  Port=35  Side=Right
  wm6 : PMIOPort  Port=36  Side=Right
  qm1 : PMIOPort  Port=37  Side=Right
  qm2 : PMIOPort  Port=38  Side=Right
  qm3 : PMIOPort  Port=39  Side=Right
  qm4 : PMIOPort  Port=40  Side=Right
  qm5 : PMIOPort  Port=41  Side=Right
  qm6 : PMIOPort  Port=42  Side=Right
  wires:
  PS-Simulink Converter/1 -> Harmonic Drive Torque/1  "joint1"
  PS-Simulink Converter1/1 -> Harmonic Drive Torque/2  "joint2"
  PS-Simulink Converter2/1 -> Harmonic Drive Torque/3  "joint3"
  PS-Simulink Converter3/1 -> Harmonic Drive Torque/4  "joint4"
  PS-Simulink Converter4/1 -> Harmonic Drive Torque/5  "joint5"
  PS-Simulink Converter5/1 -> Harmonic Drive Torque/6  "joint6"
  connections:
  wrist_2_link/LConn1 -- wrist_2_joint/RConn1
  wrist_1_joint/RConn3 -- qd4/RConn1 -- Harmonic Drive 4/RConn1
  wrist_2_link/RConn1 -- wrist_3_joint/LConn1
  shoulder_link/LConn1 -- shoulder_pan_joint/RConn1
  World/RConn1 -- Spline1/LConn1 -- world_joint/LConn1 -- Rigid Transform/RConn1 -- MechanismConfiguration/RConn1 -- Solver Configuration/RConn1
  upper_arm_link/LConn1 -- shoulder_lift_joint/RConn1
  shoulder_pan_joint/RConn2 -- q1/RConn1
  base_link/RConn1 -- shoulder_pan_joint/LConn1
  shoulder_lift_joint/RConn2 -- q2/RConn1
  ee_fixed_joint/RConn1 -- ee_link/LConn1
  wrist_2_joint/RConn3 -- qd5/RConn1 -- Harmonic Drive 5/RConn1
  wrist_3_joint/RConn2 -- q6/RConn1
  elbow_joint/RConn3 -- qd3/RConn1 -- Harmonic Drive 3/RConn1
  shoulder_link/RConn1 -- shoulder_lift_joint/LConn1
  base_link/LConn1 -- world_joint/RConn1
  elbow_joint/RConn2 -- q3/RConn1
  forearm_link/LConn1 -- elbow_joint/RConn1
  wrist_1_link/LConn1 -- wrist_1_joint/RConn1
  forearm_link/RConn1 -- wrist_1_joint/LConn1
  wrist_1_link/RConn1 -- wrist_2_joint/LConn1
  wrist_3_link/LConn1 -- wrist_3_joint/RConn1
  upper_arm_link/RConn1 -- elbow_joint/LConn1
  wrist_3_link/RConn1 -- ee_fixed_joint/LConn1
  wrist_3_joint/RConn3 -- qd6/RConn1 -- Harmonic Drive 6/RConn1
  shoulder_lift_joint/RConn3 -- Harmonic Drive 2/RConn1 -- qd2/RConn1
  wrist_2_joint/RConn2 -- q5/RConn1
  wrist_1_joint/RConn2 -- q4/RConn1
  Brick Solid/RConn1 -- Rigid Transform/LConn1
  qd1/RConn1 -- shoulder_pan_joint/RConn3 -- Harmonic Drive 1/RConn1
  Harmonic Drive 4/LConn1 -- u4/RConn1
  u6/RConn1 -- Harmonic Drive 6/LConn1
  u5/RConn1 -- Harmonic Drive 5/LConn1
  u3/RConn1 -- Harmonic Drive 3/LConn1
  u2/RConn1 -- Harmonic Drive 2/LConn1
  u1/RConn1 -- Harmonic Drive 1/LConn1
  Harmonic Drive 6/LConn2 -- PS-Simulink Converter5/LConn1 -- wrist_3_joint/LConn2
  Harmonic Drive 5/LConn2 -- wrist_2_joint/LConn2 -- PS-Simulink Converter4/LConn1
  Harmonic Drive 4/LConn2 -- PS-Simulink Converter3/LConn1 -- wrist_1_joint/LConn2
  elbow_joint/LConn2 -- PS-Simulink Converter2/LConn1 -- Harmonic Drive 3/LConn2
  Harmonic Drive 1/LConn2 -- shoulder_pan_joint/LConn2 -- PS-Simulink Converter/LConn1
  Harmonic Drive 2/LConn2 -- shoulder_lift_joint/LConn2 -- PS-Simulink Converter1/LConn1
  wl1/RConn1 -- Harmonic Drive 1/RConn2
  wl2/RConn1 -- Harmonic Drive 2/RConn2
  wl3/RConn1 -- Harmonic Drive 3/RConn2
  wl4/RConn1 -- Harmonic Drive 4/RConn2
  wl5/RConn1 -- Harmonic Drive 5/RConn2
  wl6/RConn1 -- Harmonic Drive 6/RConn2
  ql1/RConn1 -- Harmonic Drive 1/RConn3
  ql2/RConn1 -- Harmonic Drive 2/RConn3
  ql3/RConn1 -- Harmonic Drive 3/RConn3
  ql4/RConn1 -- Harmonic Drive 4/RConn3
  ql5/RConn1 -- Harmonic Drive 5/RConn3
  ql6/RConn1 -- Harmonic Drive 6/RConn3
  wm1/RConn1 -- Harmonic Drive 1/LConn3
  wm2/RConn1 -- Harmonic Drive 2/LConn3
  wm3/RConn1 -- Harmonic Drive 3/LConn3
  wm4/RConn1 -- Harmonic Drive 4/LConn3
  wm5/RConn1 -- Harmonic Drive 5/LConn3
  wm6/RConn1 -- Harmonic Drive 6/LConn3
  qm1/RConn1 -- Harmonic Drive 1/LConn4
  qm2/RConn1 -- Harmonic Drive 2/LConn4
  qm3/RConn1 -- Harmonic Drive 3/LConn4
  qm4/RConn1 -- Harmonic Drive 4/LConn4
  qm5/RConn1 -- Harmonic Drive 5/LConn4
  qm6/RConn1 -- Harmonic Drive 6/LConn4

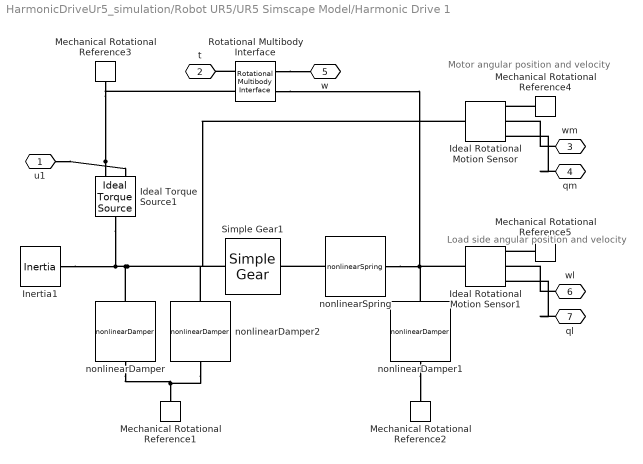
== system HarmonicDriveUr5_simulation/Robot UR5/UR5 Simscape Model/Harmonic Drive 1 ==
  note: Load side angular position and velocity
  note: Motor angular position and velocity
  Ideal Rotational Motion Sensor : fl_lib/Mechanical/Mechanical Sensors/Ideal Rotational Motion Sensor  wrap_angle=simscape.enum.onoff.off  offset=0 rad
  Ideal Rotational Motion Sensor1 : fl_lib/Mechanical/Mechanical Sensors/Ideal Rotational Motion Sensor  wrap_angle=simscape.enum.onoff.off  offset=0 rad
  Ideal Torque Source1 : fl_lib/Mechanical/Mechanical Sources/Ideal Torque Source
  Inertia1 : fl_lib/Mechanical/Rotational Elements/Inertia  inertia=1.07 kg*m^2  num_ports=foundation.enum.numPorts2.one  w_specify=off  w_priority=High  w=0 rad/s  w_nominal_specify=off  w_nominal_unit=rad/s  w_nominal_value=1  t_specify=off  t_priority=None  t=0 N*m  t_nominal_specify=off  t_nominal_unit=N*m  t_nominal_value=1
  Mechanical Rotational Reference{1..5} (5 alike) : fl_lib/Mechanical/Rotational Elements/Mechanical Rotational Reference
  Rotational Multibody Interface : fl_lib/Mechanical/Multibody Interfaces/Rotational Multibody Interface
      settings: SourceProductBaseCode=SS
  Simple Gear1 : sdl_lib/Gears/Simple Gear  ratio=100  rotation_direction=sdl.enum.shaftOutputDirection.same  friction_model=sdl.enum.gear_efficiencies_load.off  mu_visc=[0, 0] N*m/(rad/s)  T_noload=0.1 N*m  T_nom=5 N*m  efficiency_nom=0.8  efficiency=0.8  temperature_TLU=[280, 300, 320] K  load_TLU=[1, 5, 10] N*m  efficiency_TLU=[.95, .9, .85]  efficiency_TLU2=[.85, .8, .75; .95, .9, .85; .85, .8, .7]  w_thr=0.01 rad/s  pwr_thr=0.001 W  thermal_mass=50 J/K  enable_faults=simscape.enum.onoff.off  efficiency_fault=0.05  external_fault=simscape.enum.onoff.off  temporal_fault=simscape.enum.onoff.off  fault_time=5 s  fault_angles=pi / 12 rad  report_fault=simscape.enum.assert.action.none  temperature_specify=off  temperature_priority=High  temperature=300 K  temperature_nominal_specify=off  temperature_nominal_unit=K  temperature_nominal_value=1
  nonlinearDamper : CustomComponents_lib/nonlinearDamper  B=0.00064 N*m/(rad/s)  B1=0.008 N*m  B2=-0.007 N*m  t_specify=off  t_priority=None  t=0 N*m  t_nominal_specify=off  t_nominal_unit=N*m  t_nominal_value=1  w_specify=off  w_priority=None  w=0 rad/s  w_nominal_specify=off  w_nominal_unit=rad/s  w_nominal_value=1
      settings: InternalSimscapePortConfiguration="{\"Bottom\":[],\"Left\":[{\"id\":\"r\",\"label\":\"R\",\"type\":\"foundation.mechanical.rotational.rotational\"}],\"Right\":[{\"id\":\"c\",\"label\":\"C\",\"type\":\"foundation.mechanical.rotational.rotational\"}],\"Top\":[]}"
  nonlinearDamper1 : CustomComponents_lib/nonlinearDamper  B=0.00064 N*m/(rad/s)  B1=0.008 N*m  B2=-0.007 N*m  t_specify=off  t_priority=None  t=0 N*m  t_nominal_specify=off  t_nominal_unit=N*m  t_nominal_value=1  w_specify=off  w_priority=None  w=0 rad/s  w_nominal_specify=off  w_nominal_unit=rad/s  w_nominal_value=1
      settings: InternalSimscapePortConfiguration="{\"Bottom\":[],\"Left\":[{\"id\":\"r\",\"label\":\"R\",\"type\":\"foundation.mechanical.rotational.rotational\"}],\"Right\":[{\"id\":\"c\",\"label\":\"C\",\"type\":\"foundation.mechanical.rotational.rotational\"}],\"Top\":[]}"
  nonlinearDamper2 : CustomComponents_lib/nonlinearDamper  B=0.00064 N*m/(rad/s)  B1=0.008 N*m  B2=-0.007 N*m  t_specify=off  t_priority=None  t=0 N*m  t_nominal_specify=off  t_nominal_unit=N*m  t_nominal_value=1  w_specify=off  w_priority=None  w=0 rad/s  w_nominal_specify=off  w_nominal_unit=rad/s  w_nominal_value=1
      settings: InternalSimscapePortConfiguration="{\"Bottom\":[],\"Left\":[{\"id\":\"r\",\"label\":\"R\",\"type\":\"foundation.mechanical.rotational.rotational\"}],\"Right\":[{\"id\":\"c\",\"label\":\"C\",\"type\":\"foundation.mechanical.rotational.rotational\"}],\"Top\":[]}"
  nonlinearSpring : CustomComponents_lib/nonlinearSpring  K1=HFUS25.K1 N*m/rad  K2=HFUS25.K2 N*m/rad  K3=HFUS25.K3 N*m/rad  T1=HFUS25.T1 N*m  T2=HFUS25.T2 N*m  theta_specify=off  theta_priority=None  theta=0 rad  theta_nominal_specify=off  theta_nominal_unit=rad  theta_nominal_value=1  t_specify=off  t_priority=None  t=0 N*m  t_nominal_specify=off  t_nominal_unit=N*m  t_nominal_value=1  w_specify=off  w_priority=None  w=0 rad/s  w_nominal_specify=off  w_nominal_unit=rad/s  w_nominal_value=1
      settings: InternalSimscapePortConfiguration="{\"Bottom\":[],\"Left\":[{\"id\":\"r\",\"label\":\"r\",\"type\":\"foundation.mechanical.rotational.rotational\"}],\"Right\":[{\"id\":\"c\",\"label\":\"c\",\"type\":\"foundation.mechanical.rotational.rotational\"}],\"Top\":[]}"
  u1 : PMIOPort  Side=Left
  t : PMIOPort  Port=2  Side=Left
  wm : PMIOPort  Port=3  Side=Left
  qm : PMIOPort  Port=4  Side=Left
  w : PMIOPort  Port=5  Side=Right
  wl : PMIOPort  Port=6  Side=Right
  ql : PMIOPort  Port=7  Side=Right
  connections:
  Ideal Torque Source1/RConn2 -- Rotational Multibody Interface/LConn2 -- Mechanical Rotational Reference3/LConn1
  u1/RConn1 -- Ideal Torque Source1/RConn1
  Rotational Multibody Interface/LConn1 -- t/RConn1
  nonlinearSpring/LConn1 -- Simple Gear1/RConn1
  Ideal Rotational Motion Sensor/LConn1 -- Simple Gear1/LConn1 -- nonlinearDamper2/LConn1 -- nonlinearDamper/LConn1 -- Ideal Torque Source1/LConn1 -- Inertia1/LConn1
  Rotational Multibody Interface/RConn1 -- w/RConn1
  nonlinearDamper/RConn1 -- nonlinearDamper2/RConn1 -- Mechanical Rotational Reference1/LConn1
  Rotational Multibody Interface/RConn2 -- nonlinearSpring/RConn1 -- nonlinearDamper1/LConn1 -- Ideal Rotational Motion Sensor1/LConn1
  nonlinearDamper1/RConn1 -- Mechanical Rotational Reference2/LConn1
  wm/RConn1 -- Ideal Rotational Motion Sensor/RConn2
  qm/RConn1 -- Ideal Rotational Motion Sensor/RConn3
  Mechanical Rotational Reference4/LConn1 -- Ideal Rotational Motion Sensor/RConn1
  wl/RConn1 -- Ideal Rotational Motion Sensor1/RConn2
  ql/RConn1 -- Ideal Rotational Motion Sensor1/RConn3
  Mechanical Rotational Reference5/LConn1 -- Ideal Rotational Motion Sensor1/RConn1
